simulink model "c00010M_harness"  (R2018a)
settings: Solver=FixedStepAuto  StartTime=0.0  StopTime=300  FixedStep=0.1  RelTol=1e-3
undefined symbols (not defined in the file): A1, hmax, PriorityTank, R1, R2, sigbuilder_block, TempThreshold
(part 39 of 40)

== stateflow chart c00010M_harness/M176/Tank3/Control/Maintenance/Chart ==
  state InitialState
    entry: LiquidIn = 0;
    LiquidOut = 0;
  state Step1
    entry: LiquidIn = 0;
    LiquidOut = 1;
  state Step2
    entry: LiquidIn = 1;
    LiquidOut = 0;
  state Step3
    entry: LiquidIn = 0;
    LiquidOut = 0;
  (default) -> InitialState
  Step3 -> InitialState : [Type~=1||LiquidLevel <=0.01]
  Step2 -> InitialState [order 1] : [Type~=1]
  Step1 -> InitialState [order 1] : [Type ~= 1]
  InitialState -> Step1 : [StartMaintenance == 1 && Type ==1]
  Step1 -> Step2 [order 2] : [LiquidLevel <=0.01]
  Step2 -> Step3 [order 2] : [LiquidLevel>=hmax*0.9]
  data: Type input; StartMaintenance input; LiquidIn output; LiquidOut output; LiquidLevel input; hmax parameter

== stateflow chart c00010M_harness/M177/Tank3/Control/Maintenance/Chart ==
  state InitialState
    entry: LiquidIn = 0;
    LiquidOut = 0;
  state Step1
    entry: LiquidIn = 0;
    LiquidOut = 1;
  state Step2
    entry: LiquidIn = 1;
    LiquidOut = 0;
  state Step3
    entry: LiquidIn = 0;
    LiquidOut = 1;
  (default) -> InitialState
  Step3 -> InitialState : [Type~=1||LiquidLevel <=0.01]
  Step2 -> InitialState [order 1] : [Type~=1]
  InitialState -> Step1 : [StartMaintenance == 1 && Type ==1]
  Step1 -> Step2 : [LiquidLevel <=0.01]
  Step2 -> Step3 [order 2] : [LiquidLevel>=hmax*0.9]
  data: Type input; StartMaintenance input; LiquidIn output; LiquidOut output; LiquidLevel input; hmax parameter

== stateflow chart c00010M_harness/M178/Tank3/Control/Maintenance/Chart ==
  state InitialState
    entry: LiquidIn = 0;
    LiquidOut = 0;
  state Step1
    entry: LiquidIn = 0;
    LiquidOut = 1;
  state Step2
    entry: LiquidIn = 1;
    LiquidOut = 0;
  state Step3
    entry: LiquidIn = 0;
    LiquidOut = 1;
  (default) -> InitialState
  Step3 -> InitialState : [Type~=1||LiquidLevel <=0.01]
  Step1 -> InitialState [order 1] : [Type ~= 1]
  InitialState -> Step1 : [StartMaintenance == 1 && Type ==1]
  Step1 -> Step2 [order 2] : [LiquidLevel <=0.01]
  Step2 -> Step3 : [LiquidLevel>=hmax*0.9]
  data: Type input; StartMaintenance input; LiquidIn output; LiquidOut output; LiquidLevel input; hmax parameter

== stateflow chart c00010M_harness/M179/Tank3/Control/Maintenance/Chart ==
  state InitialState
    entry: LiquidIn = 0;
    LiquidOut = 0;
  state Step1
    entry: LiquidIn = 0;
    LiquidOut = 1;
  state Step2
    entry: LiquidIn = 1;
    LiquidOut = 0;
  state Step3
    entry: LiquidIn = 0;
    LiquidOut = 1;
  (default) -> InitialState
  Step3 -> InitialState : [Type~=1||LiquidLevel <=0.01]
  Step2 -> InitialState [order 1] : [Type~=1]
  Step1 -> InitialState [order 1] : [Type ~= 1]
  InitialState -> Step1 : [StartMaintenance ~= 1 && Type ==1]
  Step1 -> Step2 [order 2] : [LiquidLevel <=0.01]
  Step2 -> Step3 [order 2] : [LiquidLevel>=hmax*0.9]
  data: Type input; StartMaintenance input; LiquidIn output; LiquidOut output; LiquidLevel input; hmax parameter

== stateflow chart c00010M_harness/M180/Tank3/Control/Maintenance/Chart ==
  state InitialState
    entry: LiquidIn = 0;
    LiquidOut = 0;
  state Step1
    entry: LiquidIn = 0;
    LiquidOut = 1;
  state Step2
    entry: LiquidIn = 1;
    LiquidOut = 0;
  state Step3
    entry: LiquidIn = 0;
    LiquidOut = 1;
  (default) -> InitialState
  Step3 -> InitialState : [Type~=1||LiquidLevel <=0.01]
  Step2 -> InitialState [order 1] : [Type~=1]
  Step1 -> InitialState [order 1] : [Type == 1]
  InitialState -> Step1 : [StartMaintenance == 1 && Type ==1]
  Step1 -> Step2 [order 2] : [LiquidLevel <=0.01]
  Step2 -> Step3 [order 2] : [LiquidLevel>=hmax*0.9]
  data: Type input; StartMaintenance input; LiquidIn output; LiquidOut output; LiquidLevel input; hmax parameter

== stateflow chart c00010M_harness/M181/Tank3/Control/Maintenance/Chart ==
  state InitialState
    entry: LiquidIn = 0;
    LiquidOut = 0;
  state Step1
    entry: LiquidIn = 0;
    LiquidOut = 1;
  state Step2
    entry: LiquidIn = 1;
    LiquidOut = 0;
  state Step3
    entry: LiquidIn = 0;
    LiquidOut = 1;
  (default) -> InitialState
  Step3 -> InitialState : [Type~=1||LiquidLevel <=0.01]
  Step2 -> InitialState [order 1] : [Type~=1]
  Step1 -> InitialState [order 1] : [Type ~= 1]
  InitialState -> Step1 : [StartMaintenance == 1 && Type ==1]
  Step1 -> Step2 [order 2] : [LiquidLevel >=0.01]
  Step2 -> Step3 [order 2] : [LiquidLevel>=hmax*0.9]
  data: Type input; StartMaintenance input; LiquidIn output; LiquidOut output; LiquidLevel input; hmax parameter

== stateflow chart c00010M_harness/M182/Tank3/Control/Maintenance/Chart ==
  state InitialState
    entry: LiquidIn = 0;
    LiquidOut = 0;
  state Step1
    entry: LiquidIn = 0;
    LiquidOut = 1;
  state Step2
    entry: LiquidIn = 1;
    LiquidOut = 0;
  state Step3
    entry: LiquidIn = 0;
    LiquidOut = 1;
  (default) -> InitialState
  Step3 -> InitialState : [Type~=1||LiquidLevel <=0.01]
  Step2 -> InitialState [order 1] : [Type==1]
  Step1 -> InitialState [order 1] : [Type ~= 1]
  InitialState -> Step1 : [StartMaintenance == 1 && Type ==1]
  Step1 -> Step2 [order 2] : [LiquidLevel <=0.01]
  Step2 -> Step3 [order 2] : [LiquidLevel>=hmax*0.9]
  data: Type input; StartMaintenance input; LiquidIn output; LiquidOut output; LiquidLevel input; hmax parameter

== stateflow chart c00010M_harness/M183/Tank3/Control/Maintenance/Chart ==
  state InitialState
    entry: LiquidIn = 0;
    LiquidOut = 0;
  state Step1
    entry: LiquidIn = 0;
    LiquidOut = 1;
  state Step2
    entry: LiquidIn = 1;
    LiquidOut = 0;
  state Step3
    entry: LiquidIn = 0;
    LiquidOut = 1;
  (default) -> InitialState
  Step3 -> InitialState : [Type~=1||LiquidLevel <=0.01]
  Step2 -> InitialState [order 1] : [Type~=1]
  Step1 -> InitialState [order 1] : [Type ~= 1]
  InitialState -> Step1 : [StartMaintenance == 1 && Type ==1]
  Step1 -> Step2 [order 2] : [LiquidLevel <=0.01]
  Step2 -> Step3 [order 2] : [LiquidLevel<=hmax*0.9]
  data: Type input; StartMaintenance input; LiquidIn output; LiquidOut output; LiquidLevel input; hmax parameter

== stateflow chart c00010M_harness/M184/Tank3/Control/Maintenance/Chart ==
  state InitialState
    entry: LiquidIn = 0;
    LiquidOut = 0;
  state Step1
    entry: LiquidIn = 0;
    LiquidOut = 1;
  state Step2
    entry: LiquidIn = 1;
    LiquidOut = 0;
  state Step3
    entry: LiquidIn = 0;
    LiquidOut = 1;
  (default) -> InitialState
  Step3 -> InitialState : [Type~=1||LiquidLevel >=0.01]
  Step2 -> InitialState [order 1] : [Type~=1]
  Step1 -> InitialState [order 1] : [Type ~= 1]
  InitialState -> Step1 : [StartMaintenance == 1 && Type ==1]
  Step1 -> Step2 [order 2] : [LiquidLevel <=0.01]
  Step2 -> Step3 [order 2] : [LiquidLevel>=hmax*0.9]
  data: Type input; StartMaintenance input; LiquidIn output; LiquidOut output; LiquidLevel input; hmax parameter

== stateflow chart c00010M_harness/M185/Tank3/Control/Maintenance/Chart ==
  state InitialState
    entry: LiquidIn = 0;
    LiquidOut = 0;
  state Step1
    entry: LiquidIn = 0;
    LiquidOut = 1;
  state Step2
    entry: LiquidIn = 1;
    LiquidOut = 0;
  state Step3
    entry: LiquidIn = 0;
    LiquidOut = 1;
  (default) -> InitialState
  Step3 -> InitialState : [Type~=1||LiquidLevel <=0.01]
  Step2 -> InitialState [order 1] : [Type~=1]
  Step1 -> InitialState [order 1] : [Type ~= 1]
  InitialState -> Step1 : [StartMaintenance == 1 && Type ==2]
  Step1 -> Step2 [order 2] : [LiquidLevel <=0.01]
  Step2 -> Step3 [order 2] : [LiquidLevel>=hmax*0.9]
  data: Type input; StartMaintenance input; LiquidIn output; LiquidOut output; LiquidLevel input; hmax parameter

== stateflow chart c00010M_harness/M186/Tank3/Control/Maintenance/Chart ==
  state InitialState
    entry: LiquidIn = 0;
    LiquidOut = 0;
  state Step1
    entry: LiquidIn = 0;
    LiquidOut = 1;
  state Step2
    entry: LiquidIn = 1;
    LiquidOut = 0;
  state Step3
    entry: LiquidIn = 0;
    LiquidOut = 1;
  (default) -> InitialState
  Step3 -> InitialState : [Type~=1||LiquidLevel <=0.01]
  Step2 -> InitialState [order 1] : [Type~=1]
  Step1 -> InitialState [order 1] : [Type ~= 2]
  InitialState -> Step1 : [StartMaintenance == 1 && Type ==1]
  Step1 -> Step2 [order 2] : [LiquidLevel <=0.01]
  Step2 -> Step3 [order 2] : [LiquidLevel>=hmax*0.9]
  data: Type input; StartMaintenance input; LiquidIn output; LiquidOut output; LiquidLevel input; hmax parameter

== stateflow chart c00010M_harness/M187/Tank3/Control/Maintenance/Chart ==
  state InitialState
    entry: LiquidIn = 0;
    LiquidOut = 0;
  state Step1
    entry: LiquidIn = 0;
    LiquidOut = 1;
  state Step2
    entry: LiquidIn = 1;
    LiquidOut = 0;
  state Step3
    entry: LiquidIn = 0;
    LiquidOut = 1;
  (default) -> InitialState
  Step3 -> InitialState : [Type~=1||LiquidLevel <=0.01]
  Step2 -> InitialState [order 1] : [Type~=1]
  Step1 -> InitialState [order 1] : [Type ~= 1]
  InitialState -> Step1 : [StartMaintenance == 1 && Type ==1]
  Step1 -> Step2 [order 2] : [LiquidLevel <=0.10]
  Step2 -> Step3 [order 2] : [LiquidLevel>=hmax*0.9]
  data: Type input; StartMaintenance input; LiquidIn output; LiquidOut output; LiquidLevel input; hmax parameter

== stateflow chart c00010M_harness/M188/Tank3/Control/Maintenance/Chart ==
  state InitialState
    entry: LiquidIn = 0;
    LiquidOut = 0;
  state Step1
    entry: LiquidIn = 0;
    LiquidOut = 1;
  state Step2
    entry: LiquidIn = 1;
    LiquidOut = 0;
  state Step3
    entry: LiquidIn = 0;
    LiquidOut = 1;
  (default) -> InitialState
  Step3 -> InitialState : [Type~=1||LiquidLevel <=0.01]
  Step2 -> InitialState [order 1] : [Type~=2]
  Step1 -> InitialState [order 1] : [Type ~= 1]
  InitialState -> Step1 : [StartMaintenance == 1 && Type ==1]
  Step1 -> Step2 [order 2] : [LiquidLevel <=0.01]
  Step2 -> Step3 [order 2] : [LiquidLevel>=hmax*0.9]
  data: Type input; StartMaintenance input; LiquidIn output; LiquidOut output; LiquidLevel input; hmax parameter

== stateflow chart c00010M_harness/M189/Tank3/Control/Maintenance/Chart ==
  state InitialState
    entry: LiquidIn = 0;
    LiquidOut = 0;
  state Step1
    entry: LiquidIn = 0;
    LiquidOut = 1;
  state Step2
    entry: LiquidIn = 1;
    LiquidOut = 0;
  state Step3
    entry: LiquidIn = 0;
    LiquidOut = 1;
  (default) -> InitialState
  Step3 -> InitialState : [Type~=1||LiquidLevel <=0.01]
  Step2 -> InitialState [order 1] : [Type~=1]
  Step1 -> InitialState [order 1] : [Type ~= 1]
  InitialState -> Step1 : [StartMaintenance == 1 && Type ==1]
  Step1 -> Step2 [order 2] : [LiquidLevel <=0.01]
  Step2 -> Step3 [order 2] : [LiquidLevel>=hmax*0.5]
  data: Type input; StartMaintenance input; LiquidIn output; LiquidOut output; LiquidLevel input; hmax parameter

== stateflow chart c00010M_harness/M190/Tank3/Control/Maintenance/Chart ==
  state InitialState
    entry: LiquidIn = 0;
    LiquidOut = 0;
  state Step1
    entry: LiquidIn = 0;
    LiquidOut = 1;
  state Step2
    entry: LiquidIn = 1;
    LiquidOut = 0;
  state Step3
    entry: LiquidIn = 0;
    LiquidOut = 1;
  (default) -> InitialState
  Step3 -> InitialState : [Type~=1||LiquidLevel <=0.10]
  Step2 -> InitialState [order 1] : [Type~=1]
  Step1 -> InitialState [order 1] : [Type ~= 1]
  InitialState -> Step1 : [StartMaintenance == 1 && Type ==1]
  Step1 -> Step2 [order 2] : [LiquidLevel <=0.01]
  Step2 -> Step3 [order 2] : [LiquidLevel>=hmax*0.9]
  data: Type input; StartMaintenance input; LiquidIn output; LiquidOut output; LiquidLevel input; hmax parameter

== stateflow chart c00010M_harness/M191/Tank3/Control/Maintenance/Chart ==
  state InitialState
    entry: LiquidIn = 0;
    LiquidOut = 0;
  state Step1
    entry: LiquidIn = 0;
    LiquidOut = 1;
  state Step2
    entry: LiquidIn = 1;
    LiquidOut = 0;
  state Step3
    entry: LiquidIn = 0;
    LiquidOut = 1;
  (default) -> InitialState
  Step3 -> InitialState : [Type~=1||LiquidLevel <=0.01]
  Step2 -> InitialState [order 1] : [Type~=1]
  Step1 -> InitialState [order 1] : [Type ~= 1]
  InitialState -> Step1 : [StartMaintenance == 1 || Type ==1]
  Step1 -> Step2 [order 2] : [LiquidLevel <=0.01]
  Step2 -> Step3 [order 2] : [LiquidLevel>=hmax*0.9]
  data: Type input; StartMaintenance input; LiquidIn output; LiquidOut output; LiquidLevel input; hmax parameter

== stateflow chart c00010M_harness/M192/Tank3/Control/Maintenance/Chart ==
  state InitialState
    entry: LiquidIn = 0;
    LiquidOut = 0;
  state Step1
    entry: LiquidIn = 0;
    LiquidOut = 1;
  state Step2
    entry: LiquidIn = 1;
    LiquidOut = 0;
  state Step3
    entry: LiquidIn = 0;
    LiquidOut = 1;
  (default) -> InitialState
  Step3 -> InitialState : [Type~=1&&LiquidLevel <=0.01]
  Step2 -> InitialState [order 1] : [Type~=1]
  Step1 -> InitialState [order 1] : [Type ~= 1]
  InitialState -> Step1 : [StartMaintenance == 1 && Type ==1]
  Step1 -> Step2 [order 2] : [LiquidLevel <=0.01]
  Step2 -> Step3 [order 2] : [LiquidLevel>=hmax*0.9]
  data: Type input; StartMaintenance input; LiquidIn output; LiquidOut output; LiquidLevel input; hmax parameter

== stateflow chart c00010M_harness/M193/Tank3/Control/Maintenance/Chart ==
  state InitialState
    entry: LiquidIn = 0;
    LiquidOut = 0;
  state Step1
    entry: LiquidIn = 0;
    LiquidOut = 1;
  state Step2
    entry: LiquidIn = 1;
    LiquidOut = 0;
  state Step3
    entry: LiquidIn = 0;
    LiquidOut = 1;
  (default) -> InitialState
  Step3 -> InitialState : [Type~=1||LiquidLevel <=0.01]
  Step2 -> InitialState [order 1] : [Type~=1]
  InitialState -> Step2 : [StartMaintenance == 1 && Type ==1]
  Step1 -> InitialState [order 1] : [Type ~= 1]
  Step1 -> Step2 [order 2] : [LiquidLevel <=0.01]
  Step2 -> Step3 [order 2] : [LiquidLevel>=hmax*0.9]
  data: Type input; StartMaintenance input; LiquidIn output; LiquidOut output; LiquidLevel input; hmax parameter

== stateflow chart c00010M_harness/M194/Tank3/Control/Maintenance/Chart ==
  state InitialState
    entry: LiquidIn = 0;
    LiquidOut = 0;
  state Step1
    entry: LiquidIn = 0;
    LiquidOut = 1;
  state Step2
    entry: LiquidIn = 1;
    LiquidOut = 0;
  state Step3
    entry: LiquidIn = 0;
    LiquidOut = 1;
  (default) -> InitialState
  Step3 -> InitialState : [Type~=1||LiquidLevel <=0.01]
  Step2 -> InitialState [order 1] : [Type~=1]
  Step1 -> InitialState [order 1] : [Type ~= 1]
  InitialState -> Step1 : [StartMaintenance == 1 && Type ==1]
  Step1 -> Step3 [order 2] : [LiquidLevel <=0.01]
  Step2 -> Step3 [order 2] : [LiquidLevel>=hmax*0.9]
  data: Type input; StartMaintenance input; LiquidIn output; LiquidOut output; LiquidLevel input; hmax parameter

== stateflow chart c00010M_harness/M195/Tank3/Control/Maintenance/Chart ==
  state InitialState
    entry: LiquidIn = 0;
    LiquidOut = 0;
  state Step1
    entry: LiquidIn = 0;
    LiquidOut = 1;
  state Step2
    entry: LiquidIn = 1;
    LiquidOut = 0;
  state Step3
    entry: LiquidIn = 0;
    LiquidOut = 1;
  (default) -> InitialState
  Step3 -> InitialState : [Type~=1||LiquidLevel <=0.01]
  Step2 -> InitialState [order 1] : [Type~=1]
  Step1 -> InitialState [order 1] : [Type ~= 1]
  InitialState -> Step1 : [StartMaintenance == 1 && Type ==1]
  Step2 -> Step1 [order 2] : [LiquidLevel>=hmax*0.9]
  Step1 -> Step2 [order 2] : [LiquidLevel <=0.01]
  data: Type input; StartMaintenance input; LiquidIn output; LiquidOut output; LiquidLevel input; hmax parameter

== stateflow chart c00010M_harness/M196/Tank3/Control/Maintenance/Chart ==
  state InitialState
    entry: LiquidIn = 0;
    LiquidOut = 0;
  state Step1
    entry: LiquidIn = 0;
    LiquidOut = 1;
  state Step2
    entry: LiquidIn = 1;
    LiquidOut = 0;
  state Step3
    entry: LiquidIn = 0;
    LiquidOut = 1;
  (default) -> InitialState
  Step2 -> InitialState [order 1] : [Type~=1]
  Step1 -> InitialState [order 1] : [Type ~= 1]
  InitialState -> Step1 : [StartMaintenance == 1 && Type ==1]
  Step3 -> Step1 : [Type~=1||LiquidLevel <=0.01]
  Step1 -> Step2 [order 2] : [LiquidLevel <=0.01]
  Step2 -> Step3 [order 2] : [LiquidLevel>=hmax*0.9]
  data: Type input; StartMaintenance input; LiquidIn output; LiquidOut output; LiquidLevel input; hmax parameter

== stateflow chart c00010M_harness/M197/Tank3/Control/Maintenance/Chart ==
  state InitialState
    entry: LiquidIn = 0;
    LiquidOut = 0;
  state Step1
    entry: LiquidIn = 0;
    LiquidOut = 1;
  state Step2
    entry: LiquidIn = 1;
    LiquidOut = 0;
  state Step3
    entry: LiquidIn = 0;
    LiquidOut = 1;
  Step3 -> InitialState : [Type~=1||LiquidLevel <=0.01]
  Step2 -> InitialState [order 1] : [Type~=1]
  Step1 -> InitialState [order 1] : [Type ~= 1]
  InitialState -> Step1 : [StartMaintenance == 1 && Type ==1]
  (default) -> Step1
  Step1 -> Step2 [order 2] : [LiquidLevel <=0.01]
  Step2 -> Step3 [order 2] : [LiquidLevel>=hmax*0.9]
  data: Type input; StartMaintenance input; LiquidIn output; LiquidOut output; LiquidLevel input; hmax parameter

== stateflow chart c00010M_harness/M198/Tank3/Control/Maintenance/Chart ==
  state InitialState
    entry: LiquidIn = 0;
    LiquidOut = 0;
  state Step1
    entry: LiquidIn = 0;
    LiquidOut = 1;
  state Step2
    entry: LiquidIn = 1;
    LiquidOut = 0;
  state Step3
    entry: LiquidIn = 0;
    LiquidOut = 1;
  Step3 -> InitialState : [Type~=1||LiquidLevel <=0.01]
  Step2 -> InitialState [order 1] : [Type~=1]
  Step1 -> InitialState [order 1] : [Type ~= 1]
  InitialState -> Step1 : [StartMaintenance == 1 && Type ==1]
  Step1 -> Step2 [order 2] : [LiquidLevel <=0.01]
  (default) -> Step2
  Step2 -> Step3 [order 2] : [LiquidLevel>=hmax*0.9]
  data: Type input; StartMaintenance input; LiquidIn output; LiquidOut output; LiquidLevel input; hmax parameter

== stateflow chart c00010M_harness/M199/Tank3/Control/Maintenance/Chart ==
  state InitialState
    entry: LiquidIn = 0;
    LiquidOut = 0;
  state Step1
    entry: LiquidIn = 0;
    LiquidOut = 1;
  state Step2
    entry: LiquidIn = 1;
    LiquidOut = 0;
  state Step3
    entry: LiquidIn = 0;
    LiquidOut = 1;
  Step3 -> InitialState : [Type~=1||LiquidLevel <=0.01]
  Step2 -> InitialState [order 1] : [Type~=1]
  Step1 -> InitialState [order 1] : [Type ~= 1]
  InitialState -> Step1 : [StartMaintenance == 1 && Type ==1]
  Step1 -> Step2 [order 2] : [LiquidLevel <=0.01]
  Step2 -> Step3 [order 2] : [LiquidLevel>=hmax*0.9]
  (default) -> Step3
  data: Type input; StartMaintenance input; LiquidIn output; LiquidOut output; LiquidLevel input; hmax parameter

== stateflow chart c00010M_harness/M200/Tank3/Control/Maintenance/Chart ==
  state InitialState
    entry: LiquidIn = 0;
    LiquidOut = 0;
  state Step1
    entry: LiquidIn = 0;
    LiquidOut = 1;
  state Step2
    entry: LiquidIn = 1;
    LiquidOut = 0;
  state Step3
    entry: LiquidIn = 0;
    LiquidOut = 1;
  (default) -> InitialState
  Step3 -> InitialState : [Type~=1||LiquidLevel <=0.01]
  Step2 -> InitialState [order 1] : [Type~=1]
  Step1 -> InitialState [order 1] : [Type ~= 1]
  InitialState -> Step1 : [StartMaintenance == 1 && Type ==1]
  Step1 -> Step2 [order 2] : [LiquidLevel <=0.01]
  Step2 -> Step3 [order 2] : [LiquidLevel>=hmax*0.9]
  data: Type input; StartMaintenance input; LiquidIn output; LiquidOut output; LiquidLevel input; hmax parameter

== stateflow chart c00010M_harness/M201/Tank3/Control/Maintenance/Chart ==
  state InitialState
    entry: LiquidIn = 0;
    LiquidOut = 0;
  state Step1
    entry: LiquidIn = 0;
    LiquidOut = 1;
  state Step2
    entry: LiquidIn = 1;
    LiquidOut = 0;
  state Step3
    entry: LiquidIn = 0;
    LiquidOut = 1;
  (default) -> InitialState
  Step3 -> InitialState : [Type~=1||LiquidLevel <=0.01]
  Step2 -> InitialState [order 1] : [Type~=1]
  Step1 -> InitialState [order 1] : [Type ~= 1]
  InitialState -> Step1 : [StartMaintenance == 1 && Type ==1]
  Step1 -> Step2 [order 2] : [LiquidLevel <=0.01]
  Step2 -> Step3 [order 2] : [LiquidLevel>=hmax*0.9]
  data: Type input; StartMaintenance input; LiquidIn output; LiquidOut output; LiquidLevel input; hmax parameter

== stateflow chart c00010M_harness/M202/Tank3/Control/Maintenance/Chart ==
  state InitialState
    entry: LiquidIn = 0;
    LiquidOut = 0;
  state Step1
    entry: LiquidIn = 0;
    LiquidOut = 1;
  state Step2
    entry: LiquidIn = 1;
    LiquidOut = 0;
  state Step3
    entry: LiquidIn = 0;
    LiquidOut = 1;
  (default) -> InitialState
  Step3 -> InitialState : [Type~=1||LiquidLevel <=0.01]
  Step2 -> InitialState [order 1] : [Type~=1]
  Step1 -> InitialState [order 1] : [Type ~= 1]
  InitialState -> Step1 : [StartMaintenance == 1 && Type ==1]
  Step1 -> Step2 [order 2] : [LiquidLevel <=0.01]
  Step2 -> Step3 [order 2] : [LiquidLevel>=hmax*0.9]
  data: Type input; StartMaintenance input; LiquidIn output; LiquidOut output; LiquidLevel input; hmax parameter

== stateflow chart c00010M_harness/M203/Tank3/Control/Maintenance/Chart ==
  state InitialState
    entry: LiquidIn = 0;
    LiquidOut = 0;
  state Step1
    entry: LiquidIn = 0;
    LiquidOut = 1;
  state Step2
    entry: LiquidIn = 1;
    LiquidOut = 0;
  state Step3
    entry: LiquidIn = 0;
    LiquidOut = 1;
  (default) -> InitialState
  Step3 -> InitialState : [Type~=1||LiquidLevel <=0.01]
  Step2 -> InitialState [order 1] : [Type~=1]
  Step1 -> InitialState [order 1] : [Type ~= 1]
  InitialState -> Step1 : [StartMaintenance == 1 && Type ==1]
  Step1 -> Step2 [order 2] : [LiquidLevel <=0.01]
  Step2 -> Step3 [order 2] : [LiquidLevel>=hmax*0.9]
  data: Type input; StartMaintenance input; LiquidIn output; LiquidOut output; LiquidLevel input; hmax parameter

== stateflow chart c00010M_harness/M204/Tank3/Control/Maintenance/Chart ==
  state InitialState
    entry: LiquidIn = 0;
    LiquidOut = 0;
  state Step1
    entry: LiquidIn = 0;
    LiquidOut = 1;
  state Step2
    entry: LiquidIn = 1;
    LiquidOut = 0;
  state Step3
    entry: LiquidIn = 0;
    LiquidOut = 1;
  (default) -> InitialState
  Step3 -> InitialState : [Type~=1||LiquidLevel <=0.01]
  Step2 -> InitialState [order 1] : [Type~=1]
  Step1 -> InitialState [order 1] : [Type ~= 1]
  InitialState -> Step1 : [StartMaintenance == 1 && Type ==1]
  Step1 -> Step2 [order 2] : [LiquidLevel <=0.01]
  Step2 -> Step3 [order 2] : [LiquidLevel>=hmax*0.9]
  data: Type input; StartMaintenance input; LiquidIn output; LiquidOut output; LiquidLevel input; hmax parameter

== stateflow chart c00010M_harness/M205/Tank3/Control/Maintenance/Chart ==
  state InitialState
    entry: LiquidIn = 0;
    LiquidOut = 0;
  state Step1
    entry: LiquidIn = 0;
    LiquidOut = 1;
  state Step2
    entry: LiquidIn = 1;
    LiquidOut = 0;
  state Step3
    entry: LiquidIn = 0;
    LiquidOut = 1;
  (default) -> InitialState
  Step3 -> InitialState : [Type~=1||LiquidLevel <=0.01]
  Step2 -> InitialState [order 1] : [Type~=1]
  Step1 -> InitialState [order 1] : [Type ~= 1]
  InitialState -> Step1 : [StartMaintenance == 1 && Type ==1]
  Step1 -> Step2 [order 2] : [LiquidLevel <=0.01]
  Step2 -> Step3 [order 2] : [LiquidLevel>=hmax*0.9]
  data: Type input; StartMaintenance input; LiquidIn output; LiquidOut output; LiquidLevel input; hmax parameter

== stateflow chart c00010M_harness/M206/Tank3/Control/Maintenance/Chart ==
  state InitialState
    entry: LiquidIn = 0;
    LiquidOut = 0;
  state Step1
    entry: LiquidIn = 0;
    LiquidOut = 1;
  state Step2
    entry: LiquidIn = 1;
    LiquidOut = 0;
  state Step3
    entry: LiquidIn = 0;
    LiquidOut = 1;
  (default) -> InitialState
  Step3 -> InitialState : [Type~=1||LiquidLevel <=0.01]
  Step2 -> InitialState [order 1] : [Type~=1]
  Step1 -> InitialState [order 1] : [Type ~= 1]
  InitialState -> Step1 : [StartMaintenance == 1 && Type ==1]
  Step1 -> Step2 [order 2] : [LiquidLevel <=0.01]
  Step2 -> Step3 [order 2] : [LiquidLevel>=hmax*0.9]
  data: Type input; StartMaintenance input; LiquidIn output; LiquidOut output; LiquidLevel input; hmax parameter

== stateflow chart c00010M_harness/M207/Tank3/Control/Maintenance/Chart ==
  state InitialState
    entry: LiquidIn = 0;
    LiquidOut = 0;
  state Step1
    entry: LiquidIn = 0;
    LiquidOut = 1;
  state Step2
    entry: LiquidIn = 1;
    LiquidOut = 0;
  state Step3
    entry: LiquidIn = 0;
    LiquidOut = 1;
  (default) -> InitialState
  Step3 -> InitialState : [Type~=1||LiquidLevel <=0.01]
  Step2 -> InitialState [order 1] : [Type~=1]
  Step1 -> InitialState [order 1] : [Type ~= 1]
  InitialState -> Step1 : [StartMaintenance == 1 && Type ==1]
  Step1 -> Step2 [order 2] : [LiquidLevel <=0.01]
  Step2 -> Step3 [order 2] : [LiquidLevel>=hmax*0.9]
  data: Type input; StartMaintenance input; LiquidIn output; LiquidOut output; LiquidLevel input; hmax parameter

== stateflow chart c00010M_harness/M208/Tank3/Control/Maintenance/Chart ==
  state InitialState
    entry: LiquidIn = 0;
    LiquidOut = 0;
  state Step1
    entry: LiquidIn = 0;
    LiquidOut = 1;
  state Step2
    entry: LiquidIn = 1;
    LiquidOut = 0;
  state Step3
    entry: LiquidIn = 0;
    LiquidOut = 1;
  (default) -> InitialState
  Step3 -> InitialState : [Type~=1||LiquidLevel <=0.01]
  Step2 -> InitialState [order 1] : [Type~=1]
  Step1 -> InitialState [order 1] : [Type ~= 1]
  InitialState -> Step1 : [StartMaintenance == 1 && Type ==1]
  Step1 -> Step2 [order 2] : [LiquidLevel <=0.01]
  Step2 -> Step3 [order 2] : [LiquidLevel>=hmax*0.9]
  data: Type input; StartMaintenance input; LiquidIn output; LiquidOut output; LiquidLevel input; hmax parameter

== stateflow chart c00010M_harness/M209/Tank3/Control/Maintenance/Chart ==
  state InitialState
    entry: LiquidIn = 0;
    LiquidOut = 0;
  state Step1
    entry: LiquidIn = 0;
    LiquidOut = 1;
  state Step2
    entry: LiquidIn = 1;
    LiquidOut = 0;
  state Step3
    entry: LiquidIn = 0;
    LiquidOut = 1;
  (default) -> InitialState
  Step3 -> InitialState : [Type~=1||LiquidLevel <=0.01]
  Step2 -> InitialState [order 1] : [Type~=1]
  Step1 -> InitialState [order 1] : [Type ~= 1]
  InitialState -> Step1 : [StartMaintenance == 1 && Type ==1]
  Step1 -> Step2 [order 2] : [LiquidLevel <=0.01]
  Step2 -> Step3 [order 2] : [LiquidLevel>=hmax*0.9]
  data: Type input; StartMaintenance input; LiquidIn output; LiquidOut output; LiquidLevel input; hmax parameter

== stateflow chart c00010M_harness/M210/Tank3/Control/Maintenance/Chart ==
  state InitialState
    entry: LiquidIn = 0;
    LiquidOut = 0;
  state Step1
    entry: LiquidIn = 0;
    LiquidOut = 1;
  state Step2
    entry: LiquidIn = 1;
    LiquidOut = 0;
  state Step3
    entry: LiquidIn = 0;
    LiquidOut = 1;
  (default) -> InitialState
  Step3 -> InitialState : [Type~=1||LiquidLevel <=0.01]
  Step2 -> InitialState [order 1] : [Type~=1]
  Step1 -> InitialState [order 1] : [Type ~= 1]
  InitialState -> Step1 : [StartMaintenance == 1 && Type ==1]
  Step1 -> Step2 [order 2] : [LiquidLevel <=0.01]
  Step2 -> Step3 [order 2] : [LiquidLevel>=hmax*0.9]
  data: Type input; StartMaintenance input; LiquidIn output; LiquidOut output; LiquidLevel input; hmax parameter

== stateflow chart c00010M_harness/M211/Tank3/Control/Maintenance/Chart ==
  state InitialState
    entry: LiquidIn = 0;
    LiquidOut = 0;
  state Step1
    entry: LiquidIn = 0;
    LiquidOut = 1;
  state Step2
    entry: LiquidIn = 1;
    LiquidOut = 0;
  state Step3
    entry: LiquidIn = 0;
    LiquidOut = 1;
  (default) -> InitialState
  Step3 -> InitialState : [Type~=1||LiquidLevel <=0.01]
  Step2 -> InitialState [order 1] : [Type~=1]
  Step1 -> InitialState [order 1] : [Type ~= 1]
  InitialState -> Step1 : [StartMaintenance == 1 && Type ==1]
  Step1 -> Step2 [order 2] : [LiquidLevel <=0.01]
  Step2 -> Step3 [order 2] : [LiquidLevel>=hmax*0.9]
  data: Type input; StartMaintenance input; LiquidIn output; LiquidOut output; LiquidLevel input; hmax parameter

== stateflow chart c00010M_harness/M212/Tank3/Control/Maintenance/Chart ==
  state InitialState
    entry: LiquidIn = 0;
    LiquidOut = 0;
  state Step1
    entry: LiquidIn = 0;
    LiquidOut = 1;
  state Step2
    entry: LiquidIn = 1;
    LiquidOut = 0;
  state Step3
    entry: LiquidIn = 0;
    LiquidOut = 1;
  (default) -> InitialState
  Step3 -> InitialState : [Type~=1||LiquidLevel <=0.01]
  Step2 -> InitialState [order 1] : [Type~=1]
  Step1 -> InitialState [order 1] : [Type ~= 1]
  InitialState -> Step1 : [StartMaintenance == 1 && Type ==1]
  Step1 -> Step2 [order 2] : [LiquidLevel <=0.01]
  Step2 -> Step3 [order 2] : [LiquidLevel>=hmax*0.9]
  data: Type input; StartMaintenance input; LiquidIn output; LiquidOut output; LiquidLevel input; hmax parameter

== stateflow chart c00010M_harness/M213/Tank3/Control/Maintenance/Chart ==
  state InitialState
    entry: LiquidIn = 0;
    LiquidOut = 0;
  state Step1
    entry: LiquidIn = 0;
    LiquidOut = 1;
  state Step2
    entry: LiquidIn = 1;
    LiquidOut = 0;
  state Step3
    entry: LiquidIn = 0;
    LiquidOut = 1;
  (default) -> InitialState
  Step3 -> InitialState : [Type~=1||LiquidLevel <=0.01]
  Step2 -> InitialState [order 1] : [Type~=1]
  Step1 -> InitialState [order 1] : [Type ~= 1]
  InitialState -> Step1 : [StartMaintenance == 1 && Type ==1]
  Step1 -> Step2 [order 2] : [LiquidLevel <=0.01]
  Step2 -> Step3 [order 2] : [LiquidLevel>=hmax*0.9]
  data: Type input; StartMaintenance input; LiquidIn output; LiquidOut output; LiquidLevel input; hmax parameter

== stateflow chart c00010M_harness/M214/Tank3/Control/Maintenance/Chart ==
  state InitialState
    entry: LiquidIn = 0;
    LiquidOut = 0;
  state Step1
    entry: LiquidIn = 0;
    LiquidOut = 1;
  state Step2
    entry: LiquidIn = 1;
    LiquidOut = 0;
  state Step3
    entry: LiquidIn = 0;
    LiquidOut = 1;
  (default) -> InitialState
  Step3 -> InitialState : [Type~=1||LiquidLevel <=0.01]
  Step2 -> InitialState [order 1] : [Type~=1]
  Step1 -> InitialState [order 1] : [Type ~= 1]
  InitialState -> Step1 : [StartMaintenance == 1 && Type ==1]
  Step1 -> Step2 [order 2] : [LiquidLevel <=0.01]
  Step2 -> Step3 [order 2] : [LiquidLevel>=hmax*0.9]
  data: Type input; StartMaintenance input; LiquidIn output; LiquidOut output; LiquidLevel input; hmax parameter

== stateflow chart c00010M_harness/M215/Tank3/Control/Maintenance/Chart ==
  state InitialState
    entry: LiquidIn = 0;
    LiquidOut = 0;
  state Step1
    entry: LiquidIn = 0;
    LiquidOut = 1;
  state Step2
    entry: LiquidIn = 1;
    LiquidOut = 0;
  state Step3
    entry: LiquidIn = 0;
    LiquidOut = 1;
  (default) -> InitialState
  Step3 -> InitialState : [Type~=1||LiquidLevel <=0.01]
  Step2 -> InitialState [order 1] : [Type~=1]
  Step1 -> InitialState [order 1] : [Type ~= 1]
  InitialState -> Step1 : [StartMaintenance == 1 && Type ==1]
  Step1 -> Step2 [order 2] : [LiquidLevel <=0.01]
  Step2 -> Step3 [order 2] : [LiquidLevel>=hmax*0.9]
  data: Type input; StartMaintenance input; LiquidIn output; LiquidOut output; LiquidLevel input; hmax parameter

== stateflow chart c00010M_harness/M216/Tank3/Control/Maintenance/Chart ==
  state InitialState
    entry: LiquidIn = 0;
    LiquidOut = 0;
  state Step1
    entry: LiquidIn = 0;
    LiquidOut = 1;
  state Step2
    entry: LiquidIn = 1;
    LiquidOut = 0;
  state Step3
    entry: LiquidIn = 0;
    LiquidOut = 1;
  (default) -> InitialState
  Step3 -> InitialState : [Type~=1||LiquidLevel <=0.01]
  Step2 -> InitialState [order 1] : [Type~=1]
  Step1 -> InitialState [order 1] : [Type ~= 1]
  InitialState -> Step1 : [StartMaintenance == 1 && Type ==1]
  Step1 -> Step2 [order 2] : [LiquidLevel <=0.01]
  Step2 -> Step3 [order 2] : [LiquidLevel>=hmax*0.9]
  data: Type input; StartMaintenance input; LiquidIn output; LiquidOut output; LiquidLevel input; hmax parameter

== stateflow chart c00010M_harness/M217/Tank3/Control/Maintenance/Chart ==
  state InitialState
    entry: LiquidIn = 0;
    LiquidOut = 0;
  state Step1
    entry: LiquidIn = 0;
    LiquidOut = 1;
  state Step2
    entry: LiquidIn = 1;
    LiquidOut = 0;
  state Step3
    entry: LiquidIn = 0;
    LiquidOut = 1;
  (default) -> InitialState
  Step3 -> InitialState : [Type~=1||LiquidLevel <=0.01]
  Step2 -> InitialState [order 1] : [Type~=1]
  Step1 -> InitialState [order 1] : [Type ~= 1]
  InitialState -> Step1 : [StartMaintenance == 1 && Type ==1]
  Step1 -> Step2 [order 2] : [LiquidLevel <=0.01]
  Step2 -> Step3 [order 2] : [LiquidLevel>=hmax*0.9]
  data: Type input; StartMaintenance input; LiquidIn output; LiquidOut output; LiquidLevel input; hmax parameter

== stateflow chart c00010M_harness/M218/Tank3/Control/Maintenance/Chart ==
  state InitialState
    entry: LiquidIn = 0;
    LiquidOut = 0;
  state Step1
    entry: LiquidIn = 0;
    LiquidOut = 1;
  state Step2
    entry: LiquidIn = 1;
    LiquidOut = 0;
  state Step3
    entry: LiquidIn = 0;
    LiquidOut = 1;
  (default) -> InitialState
  Step3 -> InitialState : [Type~=1||LiquidLevel <=0.01]
  Step2 -> InitialState [order 1] : [Type~=1]
  Step1 -> InitialState [order 1] : [Type ~= 1]
  InitialState -> Step1 : [StartMaintenance == 1 && Type ==1]
  Step1 -> Step2 [order 2] : [LiquidLevel <=0.01]
  Step2 -> Step3 [order 2] : [LiquidLevel>=hmax*0.9]
  data: Type input; StartMaintenance input; LiquidIn output; LiquidOut output; LiquidLevel input; hmax parameter

== stateflow chart c00010M_harness/M219/Tank3/Control/Maintenance/Chart ==
  state InitialState
    entry: LiquidIn = 0;
    LiquidOut = 0;
  state Step1
    entry: LiquidIn = 0;
    LiquidOut = 1;
  state Step2
    entry: LiquidIn = 1;
    LiquidOut = 0;
  state Step3
    entry: LiquidIn = 0;
    LiquidOut = 1;
  (default) -> InitialState
  Step3 -> InitialState : [Type~=1||LiquidLevel <=0.01]
  Step2 -> InitialState [order 1] : [Type~=1]
  Step1 -> InitialState [order 1] : [Type ~= 1]
  InitialState -> Step1 : [StartMaintenance == 1 && Type ==1]
  Step1 -> Step2 [order 2] : [LiquidLevel <=0.01]
  Step2 -> Step3 [order 2] : [LiquidLevel>=hmax*0.9]
  data: Type input; StartMaintenance input; LiquidIn output; LiquidOut output; LiquidLevel input; hmax parameter

== stateflow chart c00010M_harness/M220/Tank3/Control/Maintenance/Chart ==
  state InitialState
    entry: LiquidIn = 0;
    LiquidOut = 0;
  state Step1
    entry: LiquidIn = 0;
    LiquidOut = 1;
  state Step2
    entry: LiquidIn = 1;
    LiquidOut = 0;
  state Step3
    entry: LiquidIn = 0;
    LiquidOut = 1;
  (default) -> InitialState
  Step3 -> InitialState : [Type~=1||LiquidLevel <=0.01]
  Step2 -> InitialState [order 1] : [Type~=1]
  Step1 -> InitialState [order 1] : [Type ~= 1]
  InitialState -> Step1 : [StartMaintenance == 1 && Type ==1]
  Step1 -> Step2 [order 2] : [LiquidLevel <=0.01]
  Step2 -> Step3 [order 2] : [LiquidLevel>=hmax*0.9]
  data: Type input; StartMaintenance input; LiquidIn output; LiquidOut output; LiquidLevel input; hmax parameter

== stateflow chart c00010M_harness/M222/Tank3/Control/Maintenance/Chart ==
  state InitialState
    entry: LiquidIn = 0;
    LiquidOut = 0;
  state Step1
    entry: LiquidIn = 0;
    LiquidOut = 1;
  state Step2
    entry: LiquidIn = 1;
    LiquidOut = 0;
  state Step3
    entry: LiquidIn = 0;
    LiquidOut = 1;
  (default) -> InitialState
  Step3 -> InitialState : [Type~=1||LiquidLevel <=0.01]
  Step2 -> InitialState [order 1] : [Type~=1]
  Step1 -> InitialState [order 1] : [Type ~= 1]
  InitialState -> Step1 : [StartMaintenance == 1 && Type ==1]
  Step1 -> Step2 [order 2] : [LiquidLevel <=0.01]
  Step2 -> Step3 [order 2] : [LiquidLevel>=hmax*0.9]
  data: Type input; StartMaintenance input; LiquidIn output; LiquidOut output; LiquidLevel input; hmax parameter

== stateflow chart c00010M_harness/M223/Tank3/Control/Maintenance/Chart ==
  state InitialState
    entry: LiquidIn = 0;
    LiquidOut = 0;
  state Step1
    entry: LiquidIn = 0;
    LiquidOut = 1;
  state Step2
    entry: LiquidIn = 1;
    LiquidOut = 0;
  state Step3
    entry: LiquidIn = 0;
    LiquidOut = 1;
  (default) -> InitialState
  Step3 -> InitialState : [Type~=1||LiquidLevel <=0.01]
  Step2 -> InitialState [order 1] : [Type~=1]
  Step1 -> InitialState [order 1] : [Type ~= 1]
  InitialState -> Step1 : [StartMaintenance == 1 && Type ==1]
  Step1 -> Step2 [order 2] : [LiquidLevel <=0.01]
  Step2 -> Step3 [order 2] : [LiquidLevel>=hmax*0.9]
  data: Type input; StartMaintenance input; LiquidIn output; LiquidOut output; LiquidLevel input; hmax parameter

== stateflow chart c00010M_harness/M224/Tank3/Control/Maintenance/Chart ==
  state InitialState
    entry: LiquidIn = 0;
    LiquidOut = 0;
  state Step1
    entry: LiquidIn = 0;
    LiquidOut = 1;
  state Step2
    entry: LiquidIn = 1;
    LiquidOut = 0;
  state Step3
    entry: LiquidIn = 0;
    LiquidOut = 1;
  (default) -> InitialState
  Step3 -> InitialState : [Type~=1||LiquidLevel <=0.01]
  Step2 -> InitialState [order 1] : [Type~=1]
  Step1 -> InitialState [order 1] : [Type ~= 1]
  InitialState -> Step1 : [StartMaintenance == 1 && Type ==1]
  Step1 -> Step2 [order 2] : [LiquidLevel <=0.01]
  Step2 -> Step3 [order 2] : [LiquidLevel>=hmax*0.9]
  data: Type input; StartMaintenance input; LiquidIn output; LiquidOut output; LiquidLevel input; hmax parameter

== stateflow chart c00010M_harness/M225/Tank3/Control/Maintenance/Chart ==
  state InitialState
    entry: LiquidIn = 0;
    LiquidOut = 0;
  state Step1
    entry: LiquidIn = 0;
    LiquidOut = 1;
  state Step2
    entry: LiquidIn = 1;
    LiquidOut = 0;
  state Step3
    entry: LiquidIn = 0;
    LiquidOut = 1;
  (default) -> InitialState
  Step3 -> InitialState : [Type~=1||LiquidLevel <=0.01]
  Step2 -> InitialState [order 1] : [Type~=1]
  Step1 -> InitialState [order 1] : [Type ~= 1]
  InitialState -> Step1 : [StartMaintenance == 1 && Type ==1]
  Step1 -> Step2 [order 2] : [LiquidLevel <=0.01]
  Step2 -> Step3 [order 2] : [LiquidLevel>=hmax*0.9]
  data: Type input; StartMaintenance input; LiquidIn output; LiquidOut output; LiquidLevel input; hmax parameter

== stateflow chart c00010M_harness/M226/Tank3/Control/Maintenance/Chart ==
  state InitialState
    entry: LiquidIn = 0;
    LiquidOut = 0;
  state Step1
    entry: LiquidIn = 0;
    LiquidOut = 1;
  state Step2
    entry: LiquidIn = 1;
    LiquidOut = 0;
  state Step3
    entry: LiquidIn = 0;
    LiquidOut = 1;
  (default) -> InitialState
  Step3 -> InitialState : [Type~=1||LiquidLevel <=0.01]
  Step2 -> InitialState [order 1] : [Type~=1]
  Step1 -> InitialState [order 1] : [Type ~= 1]
  InitialState -> Step1 : [StartMaintenance == 1 && Type ==1]
  Step1 -> Step2 [order 2] : [LiquidLevel <=0.01]
  Step2 -> Step3 [order 2] : [LiquidLevel>=hmax*0.9]
  data: Type input; StartMaintenance input; LiquidIn output; LiquidOut output; LiquidLevel input; hmax parameter

== stateflow chart c00010M_harness/M227/Tank3/Control/Maintenance/Chart ==
  state InitialState
    entry: LiquidIn = 0;
    LiquidOut = 0;
  state Step1
    entry: LiquidIn = 0;
    LiquidOut = 1;
  state Step2
    entry: LiquidIn = 1;
    LiquidOut = 0;
  state Step3
    entry: LiquidIn = 0;
    LiquidOut = 1;
  (default) -> InitialState
  Step3 -> InitialState : [Type~=1||LiquidLevel <=0.01]
  Step2 -> InitialState [order 1] : [Type~=1]
  Step1 -> InitialState [order 1] : [Type ~= 1]
  InitialState -> Step1 : [StartMaintenance == 1 && Type ==1]
  Step1 -> Step2 [order 2] : [LiquidLevel <=0.01]
  Step2 -> Step3 [order 2] : [LiquidLevel>=hmax*0.9]
  data: Type input; StartMaintenance input; LiquidIn output; LiquidOut output; LiquidLevel input; hmax parameter

== stateflow chart c00010M_harness/M228/Tank3/Control/Maintenance/Chart ==
  state InitialState
    entry: LiquidIn = 0;
    LiquidOut = 0;
  state Step1
    entry: LiquidIn = 0;
    LiquidOut = 1;
  state Step2
    entry: LiquidIn = 1;
    LiquidOut = 0;
  state Step3
    entry: LiquidIn = 0;
    LiquidOut = 1;
  (default) -> InitialState
  Step3 -> InitialState : [Type~=1||LiquidLevel <=0.01]
  Step2 -> InitialState [order 1] : [Type~=1]
  Step1 -> InitialState [order 1] : [Type ~= 1]
  InitialState -> Step1 : [StartMaintenance == 1 && Type ==1]
  Step1 -> Step2 [order 2] : [LiquidLevel <=0.01]
  Step2 -> Step3 [order 2] : [LiquidLevel>=hmax*0.9]
  data: Type input; StartMaintenance input; LiquidIn output; LiquidOut output; LiquidLevel input; hmax parameter

== stateflow chart c00010M_harness/M229/Tank3/Control/Maintenance/Chart ==
  state InitialState
    entry: LiquidIn = 0;
    LiquidOut = 0;
  state Step1
    entry: LiquidIn = 0;
    LiquidOut = 1;
  state Step2
    entry: LiquidIn = 1;
    LiquidOut = 0;
  state Step3
    entry: LiquidIn = 0;
    LiquidOut = 1;
  (default) -> InitialState
  Step3 -> InitialState : [Type~=1||LiquidLevel <=0.01]
  Step2 -> InitialState [order 1] : [Type~=1]
  Step1 -> InitialState [order 1] : [Type ~= 1]
  InitialState -> Step1 : [StartMaintenance == 1 && Type ==1]
  Step1 -> Step2 [order 2] : [LiquidLevel <=0.01]
  Step2 -> Step3 [order 2] : [LiquidLevel>=hmax*0.9]
  data: Type input; StartMaintenance input; LiquidIn output; LiquidOut output; LiquidLevel input; hmax parameter

== stateflow chart c00010M_harness/M230/Tank3/Control/Maintenance/Chart ==
  state InitialState
    entry: LiquidIn = 0;
    LiquidOut = 0;
  state Step1
    entry: LiquidIn = 0;
    LiquidOut = 1;
  state Step2
    entry: LiquidIn = 1;
    LiquidOut = 0;
  state Step3
    entry: LiquidIn = 0;
    LiquidOut = 1;
  (default) -> InitialState
  Step3 -> InitialState : [Type~=1||LiquidLevel <=0.01]
  Step2 -> InitialState [order 1] : [Type~=1]
  Step1 -> InitialState [order 1] : [Type ~= 1]
  InitialState -> Step1 : [StartMaintenance == 1 && Type ==1]
  Step1 -> Step2 [order 2] : [LiquidLevel <=0.01]
  Step2 -> Step3 [order 2] : [LiquidLevel>=hmax*0.9]
  data: Type input; StartMaintenance input; LiquidIn output; LiquidOut output; LiquidLevel input; hmax parameter

== stateflow chart c00010M_harness/M231/Tank3/Control/Maintenance/Chart ==
  state InitialState
    entry: LiquidIn = 0;
    LiquidOut = 0;
  state Step1
    entry: LiquidIn = 0;
    LiquidOut = 1;
  state Step2
    entry: LiquidIn = 1;
    LiquidOut = 0;
  state Step3
    entry: LiquidIn = 0;
    LiquidOut = 1;
  (default) -> InitialState
  Step3 -> InitialState : [Type~=1||LiquidLevel <=0.01]
  Step2 -> InitialState [order 1] : [Type~=1]
  Step1 -> InitialState [order 1] : [Type ~= 1]
  InitialState -> Step1 : [StartMaintenance == 1 && Type ==1]
  Step1 -> Step2 [order 2] : [LiquidLevel <=0.01]
  Step2 -> Step3 [order 2] : [LiquidLevel>=hmax*0.9]
  data: Type input; StartMaintenance input; LiquidIn output; LiquidOut output; LiquidLevel input; hmax parameter

== stateflow chart c00010M_harness/M232/Tank3/Control/Maintenance/Chart ==
  state InitialState
    entry: LiquidIn = 0;
    LiquidOut = 0;
  state Step1
    entry: LiquidIn = 0;
    LiquidOut = 1;
  state Step2
    entry: LiquidIn = 1;
    LiquidOut = 0;
  state Step3
    entry: LiquidIn = 0;
    LiquidOut = 1;
  (default) -> InitialState
  Step3 -> InitialState : [Type~=1||LiquidLevel <=0.01]
  Step2 -> InitialState [order 1] : [Type~=1]
  Step1 -> InitialState [order 1] : [Type ~= 1]
  InitialState -> Step1 : [StartMaintenance == 1 && Type ==1]
  Step1 -> Step2 [order 2] : [LiquidLevel <=0.01]
  Step2 -> Step3 [order 2] : [LiquidLevel>=hmax*0.9]
  data: Type input; StartMaintenance input; LiquidIn output; LiquidOut output; LiquidLevel input; hmax parameter

== stateflow chart c00010M_harness/M233/Tank3/Control/Maintenance/Chart ==
  state InitialState
    entry: LiquidIn = 0;
    LiquidOut = 0;
  state Step1
    entry: LiquidIn = 0;
    LiquidOut = 1;
  state Step2
    entry: LiquidIn = 1;
    LiquidOut = 0;
  state Step3
    entry: LiquidIn = 0;
    LiquidOut = 1;
  (default) -> InitialState
  Step3 -> InitialState : [Type~=1||LiquidLevel <=0.01]
  Step2 -> InitialState [order 1] : [Type~=1]
  Step1 -> InitialState [order 1] : [Type ~= 1]
  InitialState -> Step1 : [StartMaintenance == 1 && Type ==1]
  Step1 -> Step2 [order 2] : [LiquidLevel <=0.01]
  Step2 -> Step3 [order 2] : [LiquidLevel>=hmax*0.9]
  data: Type input; StartMaintenance input; LiquidIn output; LiquidOut output; LiquidLevel input; hmax parameter

== stateflow chart c00010M_harness/M234/Tank3/Control/Maintenance/Chart ==
  state InitialState
    entry: LiquidIn = 0;
    LiquidOut = 0;
  state Step1
    entry: LiquidIn = 0;
    LiquidOut = 1;
  state Step2
    entry: LiquidIn = 1;
    LiquidOut = 0;
  state Step3
    entry: LiquidIn = 0;
    LiquidOut = 1;
  (default) -> InitialState
  Step3 -> InitialState : [Type~=1||LiquidLevel <=0.01]
  Step2 -> InitialState [order 1] : [Type~=1]
  Step1 -> InitialState [order 1] : [Type ~= 1]
  InitialState -> Step1 : [StartMaintenance == 1 && Type ==1]
  Step1 -> Step2 [order 2] : [LiquidLevel <=0.01]
  Step2 -> Step3 [order 2] : [LiquidLevel>=hmax*0.9]
  data: Type input; StartMaintenance input; LiquidIn output; LiquidOut output; LiquidLevel input; hmax parameter

== stateflow chart c00010M_harness/M235/Tank3/Control/Maintenance/Chart ==
  state InitialState
    entry: LiquidIn = 0;
    LiquidOut = 0;
  state Step1
    entry: LiquidIn = 0;
    LiquidOut = 1;
  state Step2
    entry: LiquidIn = 1;
    LiquidOut = 0;
  state Step3
    entry: LiquidIn = 0;
    LiquidOut = 1;
  (default) -> InitialState
  Step3 -> InitialState : [Type~=1||LiquidLevel <=0.01]
  Step2 -> InitialState [order 1] : [Type~=1]
  Step1 -> InitialState [order 1] : [Type ~= 1]
  InitialState -> Step1 : [StartMaintenance == 1 && Type ==1]
  Step1 -> Step2 [order 2] : [LiquidLevel <=0.01]
  Step2 -> Step3 [order 2] : [LiquidLevel>=hmax*0.9]
  data: Type input; StartMaintenance input; LiquidIn output; LiquidOut output; LiquidLevel input; hmax parameter

== stateflow chart c00010M_harness/M236/Tank3/Control/Maintenance/Chart ==
  state InitialState
    entry: LiquidIn = 0;
    LiquidOut = 0;
  state Step1
    entry: LiquidIn = 0;
    LiquidOut = 1;
  state Step2
    entry: LiquidIn = 1;
    LiquidOut = 0;
  state Step3
    entry: LiquidIn = 0;
    LiquidOut = 1;
  (default) -> InitialState
  Step3 -> InitialState : [Type~=1||LiquidLevel <=0.01]
  Step2 -> InitialState [order 1] : [Type~=1]
  Step1 -> InitialState [order 1] : [Type ~= 1]
  InitialState -> Step1 : [StartMaintenance == 1 && Type ==1]
  Step1 -> Step2 [order 2] : [LiquidLevel <=0.01]
  Step2 -> Step3 [order 2] : [LiquidLevel>=hmax*0.9]
  data: Type input; StartMaintenance input; LiquidIn output; LiquidOut output; LiquidLevel input; hmax parameter

== stateflow chart c00010M_harness/M237/Tank3/Control/Maintenance/Chart ==
  state InitialState
    entry: LiquidIn = 0;
    LiquidOut = 0;
  state Step1
    entry: LiquidIn = 0;
    LiquidOut = 1;
  state Step2
    entry: LiquidIn = 1;
    LiquidOut = 0;
  state Step3
    entry: LiquidIn = 0;
    LiquidOut = 1;
  (default) -> InitialState
  Step3 -> InitialState : [Type~=1||LiquidLevel <=0.01]
  Step2 -> InitialState [order 1] : [Type~=1]
  Step1 -> InitialState [order 1] : [Type ~= 1]
  InitialState -> Step1 : [StartMaintenance == 1 && Type ==1]
  Step1 -> Step2 [order 2] : [LiquidLevel <=0.01]
  Step2 -> Step3 [order 2] : [LiquidLevel>=hmax*0.9]
  data: Type input; StartMaintenance input; LiquidIn output; LiquidOut output; LiquidLevel input; hmax parameter

== stateflow chart c00010M_harness/M238/Tank3/Control/Maintenance/Chart ==
  state InitialState
    entry: LiquidIn = 0;
    LiquidOut = 0;
  state Step1
    entry: LiquidIn = 0;
    LiquidOut = 1;
  state Step2
    entry: LiquidIn = 1;
    LiquidOut = 0;
  state Step3
    entry: LiquidIn = 0;
    LiquidOut = 1;
  (default) -> InitialState
  Step3 -> InitialState : [Type~=1||LiquidLevel <=0.01]
  Step2 -> InitialState [order 1] : [Type~=1]
  Step1 -> InitialState [order 1] : [Type ~= 1]
  InitialState -> Step1 : [StartMaintenance == 1 && Type ==1]
  Step1 -> Step2 [order 2] : [LiquidLevel <=0.01]
  Step2 -> Step3 [order 2] : [LiquidLevel>=hmax*0.9]
  data: Type input; StartMaintenance input; LiquidIn output; LiquidOut output; LiquidLevel input; hmax parameter

== stateflow chart c00010M_harness/M239/Tank3/Control/Maintenance/Chart ==
  state InitialState
    entry: LiquidIn = 0;
    LiquidOut = 0;
  state Step1
    entry: LiquidIn = 0;
    LiquidOut = 1;
  state Step2
    entry: LiquidIn = 1;
    LiquidOut = 0;
  state Step3
    entry: LiquidIn = 0;
    LiquidOut = 1;
  (default) -> InitialState
  Step3 -> InitialState : [Type~=1||LiquidLevel <=0.01]
  Step2 -> InitialState [order 1] : [Type~=1]
  Step1 -> InitialState [order 1] : [Type ~= 1]
  InitialState -> Step1 : [StartMaintenance == 1 && Type ==1]
  Step1 -> Step2 [order 2] : [LiquidLevel <=0.01]
  Step2 -> Step3 [order 2] : [LiquidLevel>=hmax*0.9]
  data: Type input; StartMaintenance input; LiquidIn output; LiquidOut output; LiquidLevel input; hmax parameter

== stateflow chart c00010M_harness/M240/Tank3/Control/Maintenance/Chart ==
  state InitialState
    entry: LiquidIn = 0;
    LiquidOut = 0;
  state Step1
    entry: LiquidIn = 0;
    LiquidOut = 1;
  state Step2
    entry: LiquidIn = 1;
    LiquidOut = 0;
  state Step3
    entry: LiquidIn = 0;
    LiquidOut = 1;
  (default) -> InitialState
  Step3 -> InitialState : [Type~=1||LiquidLevel <=0.01]
  Step2 -> InitialState [order 1] : [Type~=1]
  Step1 -> InitialState [order 1] : [Type ~= 1]
  InitialState -> Step1 : [StartMaintenance == 1 && Type ==1]
  Step1 -> Step2 [order 2] : [LiquidLevel <=0.01]
  Step2 -> Step3 [order 2] : [LiquidLevel>=hmax*0.9]
  data: Type input; StartMaintenance input; LiquidIn output; LiquidOut output; LiquidLevel input; hmax parameter

== stateflow chart c00010M_harness/M241/Tank3/Control/Maintenance/Chart ==
  state InitialState
    entry: LiquidIn = 0;
    LiquidOut = 0;
  state Step1
    entry: LiquidIn = 0;
    LiquidOut = 1;
  state Step2
    entry: LiquidIn = 1;
    LiquidOut = 0;
  state Step3
    entry: LiquidIn = 0;
    LiquidOut = 1;
  (default) -> InitialState
  Step3 -> InitialState : [Type~=1||LiquidLevel <=0.01]
  Step2 -> InitialState [order 1] : [Type~=1]
  Step1 -> InitialState [order 1] : [Type ~= 1]
  InitialState -> Step1 : [StartMaintenance == 1 && Type ==1]
  Step1 -> Step2 [order 2] : [LiquidLevel <=0.01]
  Step2 -> Step3 [order 2] : [LiquidLevel>=hmax*0.9]
  data: Type input; StartMaintenance input; LiquidIn output; LiquidOut output; LiquidLevel input; hmax parameter

== stateflow chart c00010M_harness/M242/Tank3/Control/Maintenance/Chart ==
  state InitialState
    entry: LiquidIn = 0;
    LiquidOut = 0;
  state Step1
    entry: LiquidIn = 0;
    LiquidOut = 1;
  state Step2
    entry: LiquidIn = 1;
    LiquidOut = 0;
  state Step3
    entry: LiquidIn = 0;
    LiquidOut = 1;
  (default) -> InitialState
  Step3 -> InitialState : [Type~=1||LiquidLevel <=0.01]
  Step2 -> InitialState [order 1] : [Type~=1]
  Step1 -> InitialState [order 1] : [Type ~= 1]
  InitialState -> Step1 : [StartMaintenance == 1 && Type ==1]
  Step1 -> Step2 [order 2] : [LiquidLevel <=0.01]
  Step2 -> Step3 [order 2] : [LiquidLevel>=hmax*0.9]
  data: Type input; StartMaintenance input; LiquidIn output; LiquidOut output; LiquidLevel input; hmax parameter

== stateflow chart c00010M_harness/M243/Tank3/Control/Maintenance/Chart ==
  state InitialState
    entry: LiquidIn = 0;
    LiquidOut = 0;
  state Step1
    entry: LiquidIn = 0;
    LiquidOut = 1;
  state Step2
    entry: LiquidIn = 1;
    LiquidOut = 0;
  state Step3
    entry: LiquidIn = 0;
    LiquidOut = 1;
  (default) -> InitialState
  Step3 -> InitialState : [Type~=1||LiquidLevel <=0.01]
  Step2 -> InitialState [order 1] : [Type~=1]
  Step1 -> InitialState [order 1] : [Type ~= 1]
  InitialState -> Step1 : [StartMaintenance == 1 && Type ==1]
  Step1 -> Step2 [order 2] : [LiquidLevel <=0.01]
  Step2 -> Step3 [order 2] : [LiquidLevel>=hmax*0.9]
  data: Type input; StartMaintenance input; LiquidIn output; LiquidOut output; LiquidLevel input; hmax parameter

== stateflow chart c00010M_harness/M244/Tank3/Control/Maintenance/Chart ==
  state InitialState
    entry: LiquidIn = 0;
    LiquidOut = 0;
  state Step1
    entry: LiquidIn = 0;
    LiquidOut = 1;
  state Step2
    entry: LiquidIn = 1;
    LiquidOut = 0;
  state Step3
    entry: LiquidIn = 0;
    LiquidOut = 1;
  (default) -> InitialState
  Step3 -> InitialState : [Type~=1||LiquidLevel <=0.01]
  Step2 -> InitialState [order 1] : [Type~=1]
  Step1 -> InitialState [order 1] : [Type ~= 1]
  InitialState -> Step1 : [StartMaintenance == 1 && Type ==1]
  Step1 -> Step2 [order 2] : [LiquidLevel <=0.01]
  Step2 -> Step3 [order 2] : [LiquidLevel>=hmax*0.9]
  data: Type input; StartMaintenance input; LiquidIn output; LiquidOut output; LiquidLevel input; hmax parameter
